simulink model "AS_TestModel"  (R2022a)
settings: Solver=VariableStepAuto  StartTime=0.0  StopTime=10.0  FixedStep=0.001  MinStep=0.1  RelTol=1
settings Model: DataDictionary=AS_DataDictionary.sldd  Creator=CSN-Simulation  LastModifiedBy=FUGAZI
settings SolverCC: MaxConsecutiveMinStep=500  ZeroCrossAlgorithm=Adaptive
settings DataIOCC: Refine=2
settings DebuggingCC: AlgebraicLoopMsg=none  MaskedZcDiagnostic=none  IgnoredZcDiagnostic=none  InheritedTsInSrcMsg=none  UnconnectedInputMsg=warning  UnconnectedOutputMsg=warning  UnconnectedLineMsg=warning
settings RTWCC: DLArmComputeVersion=19.05

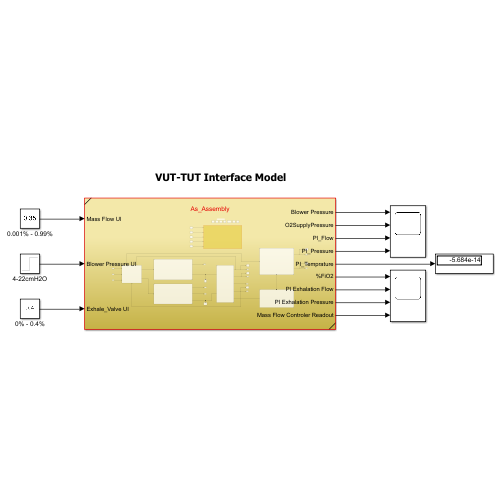
[thumbnail: Simulink's stored preview of the top-level diagram]
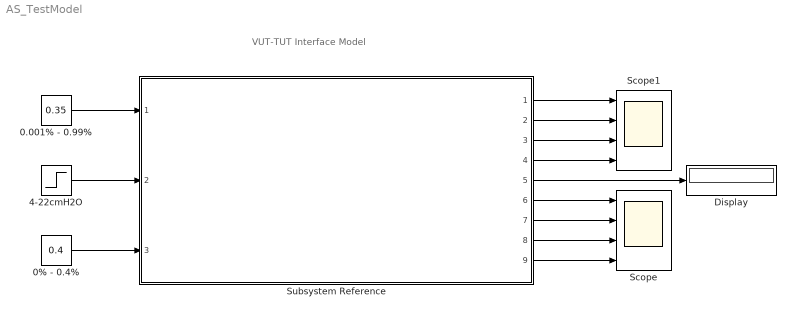
== system AS_TestModel ==
  note: VUT-TUT Interface Model
  0% - 0.4% : Constant  Value=0.4
  0.001% - 0.99% : Constant  Value=0.35
  4-22cmH2O : Step  Time=5  Before=4  After=12  SampleTime=1
  Display : Display
  Scope : Scope  NumInputPorts=4
  Scope1 : Scope  NumInputPorts=4
  Subsystem Reference : Subsystem  ReferencedSubsystem=As_Assembly
  wires:
  0.001% - 0.99%/1 -> Subsystem Reference/1
  Subsystem Reference/6 -> Scope/1
  Subsystem Reference/7 -> Scope/2
  Subsystem Reference/8 -> Scope/3
  Subsystem Reference/9 -> Scope/4
  Subsystem Reference/4 -> Scope1/4
  Subsystem Reference/3 -> Scope1/3
  Subsystem Reference/2 -> Scope1/2
  Subsystem Reference/1 -> Scope1/1
  4-22cmH2O/1 -> Subsystem Reference/2
  0% - 0.4%/1 -> Subsystem Reference/3
  Subsystem Reference/5 -> Display/1
